simulink model "D1"  (R2025b)
settings: Solver=VariableStepAuto  StartTime=0.0  StopTime=40  RelTol=1e-3
values from neighbouring files (symbols this model uses):
  T = 0.01    [D1.m]    (also in D1_param.m)
undefined symbols (not defined in the file or in its folder): Kd, Ki, Kp, umax
libraries: simulink x1
settings Model: Creator=rapaja  LastModifiedBy=Predrag
settings SolverCC: AlgebraicLoopSolver=TrustRegion
settings DebuggingCC: UnconnectedInputMsg=warning  UnconnectedOutputMsg=warning  UnconnectedLineMsg=warning
settings ModelReferenceCC: EnableRefExpFcnMdlSchedulingChecks=on
settings RTWCC: GPUComputeCapability=3.5

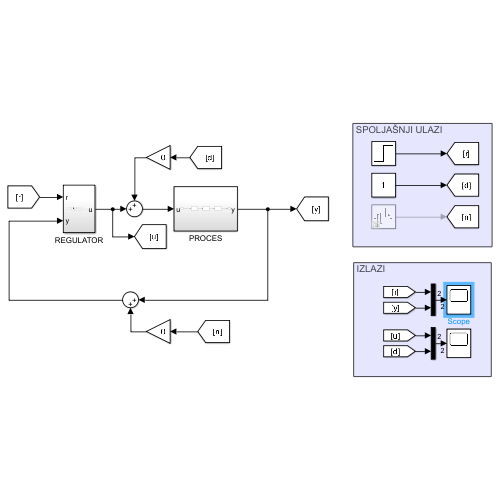
[thumbnail: Simulink's stored preview of the top-level diagram]
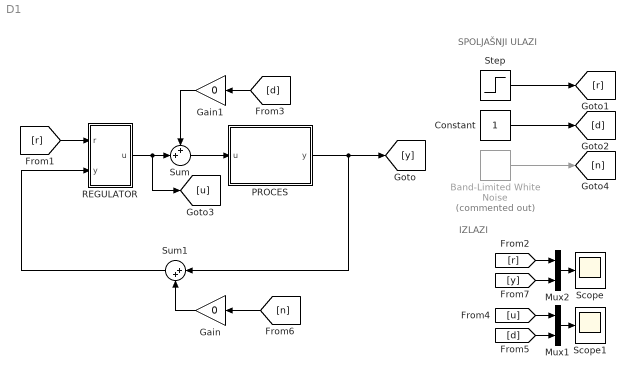
== system D1 ==
  note: IZLAZI
  note: SPOLJAŠNJI ULAZI
  Band-Limited White Noise : simulink/Sources/Band-Limited White Noise  Commented=on  Cov=[0.00001]  Ts=T  seed=[23341]
  Constant : Constant
  Gain : Gain  Gain=0
  Gain1 : Gain  Gain=0
  Mux1 : Mux  Inputs=2
  Mux2 : Mux  Inputs=2
  PROCES : Subsystem
  REGULATOR : Subsystem
  Scope : Scope
      settings: ActiveDisplayYMinimum=-3.7917033550607941  ActiveDisplayYMaximum=4.417355118428727
  Scope1 : Scope
      settings: ActiveDisplayYMinimum=-20.230336421025438  ActiveDisplayYMaximum=21.025074193059176
  Step : Step  SampleTime=0
  Sum : Sum  Inputs=++|
  Sum1 : Sum  Inputs=|++
  wires:
  Sum/1 -> PROCES/1(u)
  [r] -> REGULATOR/1(r)
  Sum1/1 -> REGULATOR/2(y)
  REGULATOR/1(u) -> [u], Sum/2
  [d] -> Gain1/1
  PROCES/1(y) -> Sum1/1, [y]
  Band-Limited White Noise/1 -> [n]
  [n] -> Gain/1
  Gain/1 -> Sum1/2
  Gain1/1 -> Sum/1
  Constant/1 -> [d]
  Step/1 -> [r]
  [r] -> Mux2/1
  [y] -> Mux2/2
  Mux2/1 -> Scope/1
  Mux1/1 -> Scope1/1
  [u] -> Mux1/1
  [d] -> Mux1/2

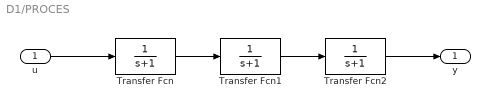
== system D1/PROCES ==
  u : Inport
  Transfer Fcn : TransferFcn  Denominator=[1 1]
  Transfer Fcn1 : TransferFcn  Denominator=[1 1]
  Transfer Fcn2 : TransferFcn  Denominator=[1 1]
  y : Outport
  wires:
  u/1 -> Transfer Fcn/1
  Transfer Fcn1/1 -> Transfer Fcn2/1
  Transfer Fcn/1 -> Transfer Fcn1/1
  Transfer Fcn2/1 -> y/1

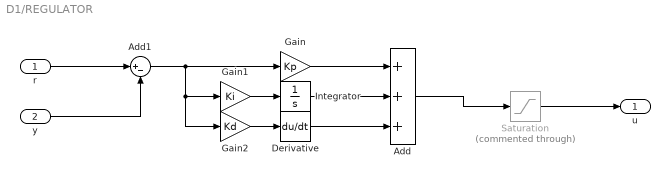
== system D1/REGULATOR ==
  r : Inport
  y : Inport  Port=2
  Add : Sum  Inputs=+++
  Add1 : Sum  Inputs=|+-
  Derivative : Derivative
  Gain : Gain  Gain=Kp
  Gain1 : Gain  Gain=Ki
  Gain2 : Gain  Gain=Kd
  Integrator : Integrator
  Saturation : Saturate  Commented=through  UpperLimit=umax  LowerLimit=-umax
  u : Outport
  wires:
  r/1 -> Add1/1
  y/1 -> Add1/2
  Gain/1 -> Add/1
  Gain1/1 -> Integrator/1
  Integrator/1 -> Add/2
  Add1/1 -> Gain/1, Gain2/1, Gain1/1
  Add/1 -> Saturation/1
  Saturation/1 -> u/1
  Gain2/1 -> Derivative/1
  Derivative/1 -> Add/3
